simulink model "c166_serial_io"  (Simulink 6.0)
settings: Solver=FixedStepDiscrete  StartTime=0.0  StopTime=inf  FixedStep=0.1  RelTol=1e-3
PreLoadFcn:
  | RTWConfigurationCB('preloadfcn', bdroot);
  | 
  | headerText = ['Embedded Target for Infineon C166' 174 ' Microcontrollers'+0 13 10];
InitFcn:
  | % START RTW CONFIGURATION CODE %
  | RTWConfigurationCB('rtw_target_initfcn',gcs);
  | % END RTW CONFIGURATION CODE %
libraries: simulink x11, c166drivers x3
settings Model: Creator=The MathWorks Inc.  LastModifiedBy=batserve  ExtModeAutoUpdateStatusClock=off  BufferReuse=off  ProdHWDeviceType=Infineon C16x
settings DataIOCC: SignalLoggingName=sigsOut
settings OptimizationCC: InlineParams=on  InlineInvariantSignals=off  OptimizeBlockIOStorage=off  BufferReuse=off  EnforceIntegerDowncast=off  ExpressionFolding=off  FoldNonRolledExpr=off  LocalBlockOutputs=off  ZeroExternalMemoryAtStartup=off  ZeroInternalMemoryAtStartup=off  InitFltsAndDblsToZero=off  LifeSpan=1
settings DebuggingCC: CheckExecutionContextPreStartOutputMsg=on  CheckExecutionContextRuntimeOutputMsg=on  SolverPrmCheckMsg=none
settings HardwareCC: ProdBitPerInt=16  ProdEndianess=LittleEndian  ProdWordSize=16  ProdHWDeviceType=Infineon C16x  TargetHWDeviceType=32-bit Generic
settings RTWCC: SystemTargetFile=c166.tlc  TemplateMakefile=c166.tmf  ProcessScript=c166_make_rtw_hook
settings CodeAppCC: IgnoreCustomStorageClasses=off
settings STFCustomTargetCC: TargetFcnLib=ansi_tfl_tmw.mat  GenFloatMathFcnCalls=ANSI_C  GenerateSampleERTMain=on  IncludeMdlTerminateFcn=off  CombineOutputUpdateFcns=on  ERTCustomFileBanners=on  SupportNonFinite=off  SupportComplex=off  PurelyIntegerCode=on  SystemTargetFile=c166.tlc
settings ERTTargetCC: TargetFcnLib=ansi_tfl_tmw.mat  GenFloatMathFcnCalls=ANSI_C  GenerateSampleERTMain=on  IncludeMdlTerminateFcn=off  SupportNonFinite=off  SupportComplex=off  PurelyIntegerCode=on  SupportContinuousTime=on  SupportNonInlinedSFcns=on  RootIOFormat=Individual Arguments  ERTCustomFileTemplate=example_file_process.tlc  InitialValueSource=Model
settings CustomProperty: DataType=RTWOptions_EnumType__toolbox_rtw_targets_c166_c166_c166_BuildActionC166  Value=Download_and_run
settings EnumStrPairs: String=Run_with_simulator

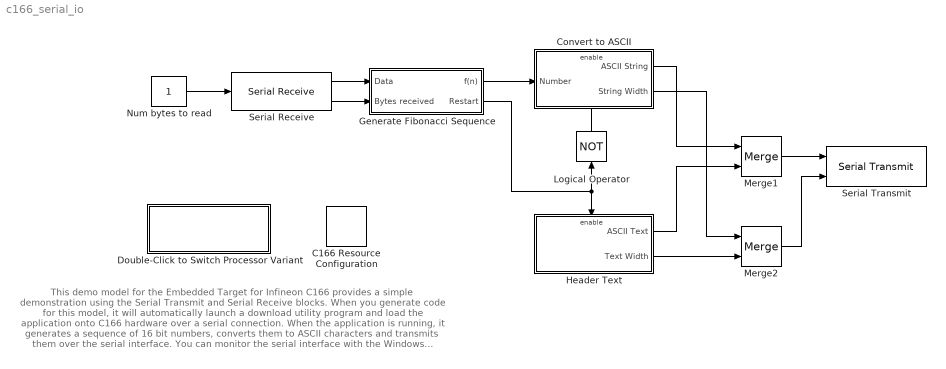
== system c166_serial_io ==
  note: This demo model for the Embedded Target for Infineon C166 provides a simple demonstration
      | using the Serial Transmit and Serial Receive blocks.
      |
      | When you generate code for this model, it will automatically launch a download utility program
      | and load the application onto C166 hardware over a serial connection. When the application is
      | running, it generates a sequence of 16 bit numbers, converts them to ASCII characters and
      | transmits them over the serial interface. You can monitor the serial interface with the Windows
      | application HyperTerminal or with the the MiniMon download utility.
      |
      | If you enter the character 'r' in the MiniMon command line field the application will restart at the
      | beginning of the sequence.
  C166 Resource Configuration : c166drivers/C166 Resource Configuration  Tag=RTW CONFIGURATION BLOCK  oldParentName=c166_serial_io  oldBlockName=|  defaultConfigLibrary=c166drivers
      | c166_serial_io/C166
      | Resource
      | Configuration
  Convert to ASCII : Subsystem  PropExecContextAcrossSSBoundary=on
  Double-Click to Switch Processor Variant : Subsystem  PropExecContextAcrossSSBoundary=on
      settings: OpenFcn=c166switchconfig(gcs)
      mask Display: disp('Switch Target\nProcessor Variant');
  Generate Fibonacci Sequence : Subsystem  PropExecContextAcrossSSBoundary=on
  Header Text : Subsystem  PropExecContextAcrossSSBoundary=on
  Logical Operator : Logic  Orientation=up  Operator=NOT  AllPortsSameDT=off
  Merge1 : Merge  AllowUnequalInputPortWidths=on
  Merge2 : Merge  AllowUnequalInputPortWidths=on
  Num bytes to read : Constant  OutDataTypeMode=uint8
  Serial Receive : c166drivers/Asynchronous//Synchronous Serial Interface/Serial Receive  show_length=on  show_bytes_read=on  max_length=1  T=0.5
  Serial Transmit : c166drivers/Asynchronous//Synchronous Serial Interface/Serial Transmit  show_length=on  show_num_sent=off  T=-1
  wires:
  Generate Fibonacci Sequence/1(f(n)) -> Convert to ASCII/1(Number)
  Generate Fibonacci Sequence/2(Restart) -> Header Text/Enable, Logical Operator/1
  Logical Operator/1 -> Convert to ASCII/Enable
  Convert to ASCII/1(ASCII String) -> Merge1/1
  Header Text/1(ASCII Text) -> Merge1/2
  Merge1/1 -> Serial Transmit/1
  Convert to ASCII/2("String Width ") -> Merge2/1
  Merge2/1 -> Serial Transmit/2
  Header Text/2(Text Width) -> Merge2/2
  Num bytes to read/1 -> Serial Receive/1
  Serial Receive/1 -> Generate Fibonacci Sequence/1(Data)
  Serial Receive/2 -> Generate Fibonacci Sequence/2(Bytes received)

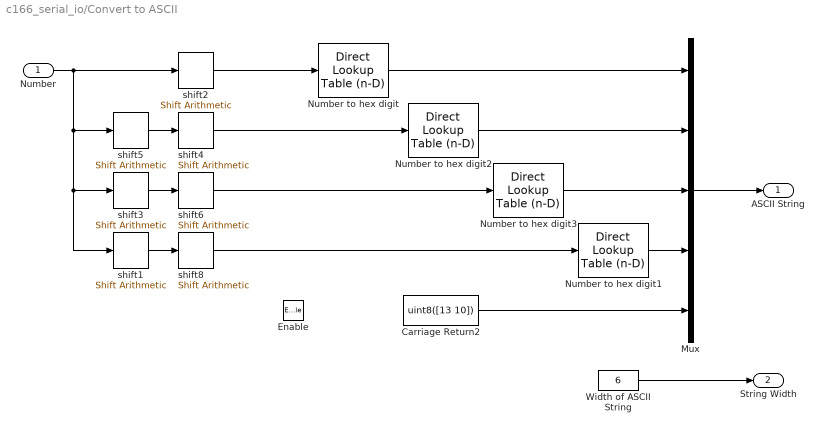
== system c166_serial_io/Convert to ASCII ==
  Number : Inport  Port=1  LatchInput=off
  Enable : EnablePort
  Carriage Return2 : Constant  Value=uint8([13 10])
  Mux : Mux  Inputs=5
  Number to hex digit{,1..3} (4 alike) : simulink/Lookup Tables/Direct Lookup Table (n-D)  maskTabDims=1  explicitNumDims=1  outDims=Element  tabIsInput=off  mxTable=uint8([48 49 50 51 52 53 54 55 56 57 65 66 67 68 69 70])  clipFlag=Warning
  Width of ASCII String : Constant  Value=6  OutDataTypeMode=uint8
  shift1 : simulink/Logic and Bit Operations/Shift Arithmetic  nBitShiftRight=-(12)  nBinPtShiftRight=0
  shift{2,4,6,8} (4 alike) : simulink/Logic and Bit Operations/Shift Arithmetic  nBitShiftRight=12  nBinPtShiftRight=0
  shift3 : simulink/Logic and Bit Operations/Shift Arithmetic  nBitShiftRight=-(8)  nBinPtShiftRight=0
  shift5 : simulink/Logic and Bit Operations/Shift Arithmetic  nBitShiftRight=-(4)  nBinPtShiftRight=0
  ASCII String : Outport  InitialOutput=[0 0 0 0 0 0]
  "String Width " : Outport  Port=2  InitialOutput=0
  wires:
  shift5/1 -> shift4/1
  shift3/1 -> shift6/1
  Number/1 -> shift2/1, shift5/1, shift3/1, shift1/1
  shift2/1 -> Number to hex digit/1
  shift4/1 -> Number to hex digit2/1
  shift6/1 -> Number to hex digit3/1
  shift8/1 -> Number to hex digit1/1
  Number to hex digit/1 -> Mux/1
  Number to hex digit2/1 -> Mux/2
  Number to hex digit3/1 -> Mux/3
  Number to hex digit1/1 -> Mux/4
  Carriage Return2/1 -> Mux/5
  shift1/1 -> shift8/1
  Mux/1 -> ASCII String/1
  Width of ASCII String/1 -> "String Width "/1

== system c166_serial_io/Double-Click to Switch Processor Variant ==

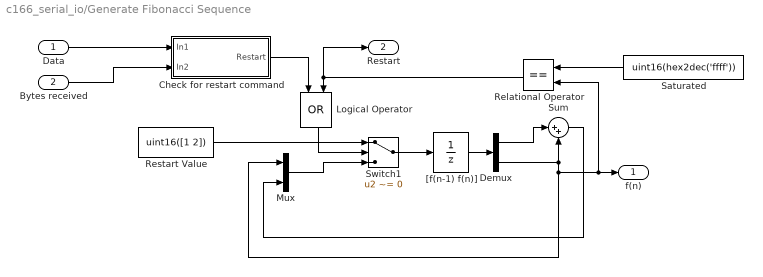
== system c166_serial_io/Generate Fibonacci Sequence ==
  Data : Inport  Port=1  LatchInput=off
  Bytes received : Inport  Port=2  LatchInput=off
  Check for restart command : Subsystem  PropExecContextAcrossSSBoundary=on
  Demux : Demux  Outputs=2
  Logical Operator : Logic  Orientation=down  Operator=OR  AllPortsSameDT=off
  Mux : Mux  Inputs=2
  Relational Operator : RelationalOperator  Orientation=left  Operator===
  Restart Value : Constant  Value=uint16([1 2])
  Saturated : Constant  Orientation=left  Value=uint16(hex2dec('ffff'))
  Sum : Sum  Inputs=|++  SaturateOnIntegerOverflow=on
  Switch1 : Switch  Criteria=u2 ~= 0  SaturateOnIntegerOverflow=on
  "[f(n-1) f(n)]" : UnitDelay  X0=uint16( [ hex2dec('ffff') hex2dec('ffff') ] )  SampleTime=0.5
  f(n) : Outport
  Restart : Outport  Port=2
  wires:
  Saturated/1 -> Relational Operator/1
  Relational Operator/1 -> Restart/1, Logical Operator/2
  Restart Value/1 -> Switch1/1
  "[f(n-1) f(n)]"/1 -> Demux/1
  Demux/1 -> Sum/1
  Switch1/1 -> "[f(n-1) f(n)]"/1
  Mux/1 -> Switch1/3
  Demux/2 -> Sum/2, Mux/1, Relational Operator/2, f(n)/1
  Sum/1 -> Mux/2
  Logical Operator/1 -> Switch1/2
  Check for restart command/1(Restart) -> Logical Operator/1
  Data/1 -> Check for restart command/1(In1)
  Bytes received/1 -> Check for restart command/2(In2)

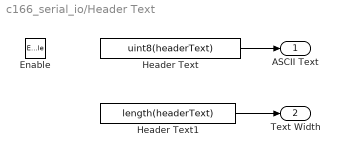
== system c166_serial_io/Header Text ==
  Enable : EnablePort
  Header Text : Constant  Value=uint8(headerText)
  Header Text1 : Constant  Value=length(headerText)  OutDataTypeMode=uint8
  ASCII Text : Outport  InitialOutput=zeros(size(headerText))
  Text Width : Outport  Port=2  InitialOutput=0
  wires:
  Header Text/1 -> ASCII Text/1
  Header Text1/1 -> Text Width/1

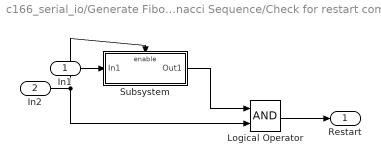
== system c166_serial_io/Generate Fibonacci Sequence/Check for restart command ==
  In1 : Inport  Port=1  LatchInput=off
  In2 : Inport  Port=2  LatchInput=off
  Logical Operator : Logic  AllPortsSameDT=off
  Subsystem : Subsystem  PropExecContextAcrossSSBoundary=on
  Restart : Outport
  wires:
  In2/1 -> Logical Operator/2, Subsystem/Enable
  Logical Operator/1 -> Restart/1
  Subsystem/1(Out1) -> Logical Operator/1
  In1/1 -> Subsystem/1(In1)

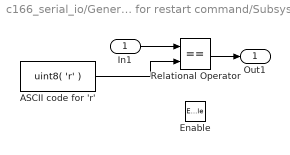
== system c166_serial_io/Generate Fibonacci Sequence/Check for restart command/Subsystem ==
  In1 : Inport  Port=1  LatchInput=off
  Enable : EnablePort
  ASCII code for 'r' : Constant  Value=uint8( 'r' )
  Relational Operator : RelationalOperator  Operator===
  Out1 : Outport
  wires:
  ASCII code for 'r'/1 -> Relational Operator/2
  In1/1 -> Relational Operator/1
  Relational Operator/1 -> Out1/1
